simulink model "hd"  (R2016b)
settings: Solver=VariableStepAuto  StartTime=0.0  StopTime=totaltime  RelTol=1e-3
undefined symbols (not defined in the file or in its folder): A, N, st
libraries: xbsIndex_r4 x1, JTAGRuntimeCosim_r4 x1
settings Model: Creator=rm101  LastModifiedBy=rm101

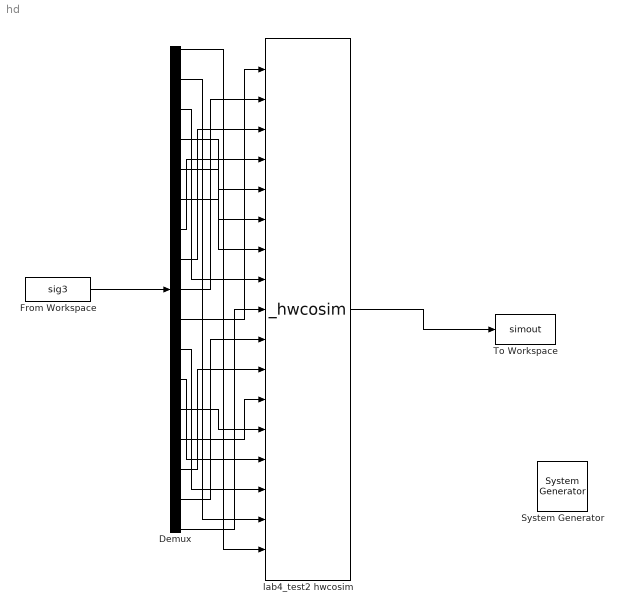
== system hd ==
  " System Generator" : xbsIndex_r4/ System Generator  Tag=genX  xilinxfamily=zynq  part=xc7z020  speed=-1  package=clg484  synthesis_tool=Vivado  clock_wrapper=Clock Enables  directory=C:/Users/rm101/Desktop/YG/Lab4_Matlab/gen  proj_type=Vivado  Synth_file=Vivado Synthesis Defaults  Impl_file=Vivado Implementation Defaults  testbench=off  simulink_period=st  sysclk_period=st*10e8  dcm_input_clock_period=10  incr_netlist=off  trim_vbits=Everywhere in SubSystem  dbl_ovrd=According to Block Masks  core_generation=According to Block Masks  run_coregen=off  deprecated_control=off  eval_field=0  block_type=sysgen
  Demux : Demux  Outputs=17
  From Workspace : FromWorkspace  VariableName=sig3  SampleTime=0  Interpolate=off  OutputAfterFinalValue=Holding final value
  To Workspace : ToWorkspace  VariableName=simout  SaveFormat=Timeseries  SampleTime=-1
  lab4_test2 hwcosim : JTAGRuntimeCosim_r4/_hwcosim  clkSrc=Single Stepped  hasCombinationalPath=on  bitfileName=C:\Users\rm101\Desktop\YG\Lab4_Matlab\gen\lab4_test2.bit  skipConfig=off  dispPartInfo=off  useZynqReconfigScript=on  cable=Auto Detect  speed=N/A  cablePort=N/A  cableLocation=Local  shareCable=off  design_xtable=|  engineDll=JTAGCosimEngine.dll  cableWaitTime=10  bscanPos=-1  IRLengths=[]  useWaitBox=1  hasBufgmux=on  Scheme=Cosim  useCmdProc=1  hasProc=0  useImpact=0  printLogFile=0  userChain=2  block_type=jtagcosim
      | {
      |     'clkWrapper' => 'lab4_test2',
      |     'burstMode' => false,
      |     'burstFifoDepth' => '1024',
      |     'shared_memories' => {},
      |     'clocksGcd' => 1,
      |     'device' => {
      |       'family' => 'zynq',
      |       'part' => 'xc7z020',
      |       'package' => 'clg484',
      |       'speed' => '-1',
      |     },
      |     'ports' => {
      |       'a9' => {
      |         'direction' => 'in',
      |         'width' => 8,
      |         'name' => 'a9',
      |         'period' => 1,
      |         'icon_text' => 'a9',
      |         'type' => 'Fix_8_6',
      |         'arithmetic_type' => 'xlSigned',
      |         'dat_file' => 'lab4_test2_subsystem_a9.dat',
      |         'bin_pt' => 6,
      |         'addr_offset' => 0,
      |         'bd_port_index' => 0,
      |       },
      |       'a8' => {
      |         'direction' => 'in',
      |         'width' => 8,
      |         'name' => 'a8',
      |         'period' => 1,
      |         'icon_text' => 'a8',
      |         'type' => 'Fix_8_6',
      |         'arithmetic_type' => 'xlSigned',
      |         'dat_file' => 'lab4_test2_subsystem_a8.dat',
      |         'bin_pt' => 6,
      |         'addr_offset' => 4,
      |         'bd_port_index' => 1,
      |       },
      |       'a7' => {
      |         'direction' => 'in',
      |         'width' => 8,
      |         'name' => 'a7',
      |         'period' => 1,
      |         'icon_text' => 'a7',
      |         'type' => 'Fix_8_6',
      |         'arithmetic_type' => 'xlSigned',
      |         'dat_file' => 'lab4_test2_subsystem_a7.dat',
      |         'bin_pt' => 6,
      |         'addr_offset' => 8,
      |         'bd_port_index' => 2,
      |       },
      |       'a6' => {
      |         'direction' => 'in',
      |         'width' => 8,
      |         'name' => 'a6',
      |         'period' => 1,
      |         'icon_text' => 'a6',
      |         'type' => 'Fix_8_6',
      |         'arithmetic_type' => 'xlSigned',
      |         'dat_file' => 'lab4_test2_subsystem_a6.dat',
      |         'bin_pt' => 6,
      |         'addr_offset' => 12,
      |         'bd_port_index' => 3,
      |       },
      |       'a5' => {
      |         'direction' => 'in',
      |         'width' => 8,
      |         'name' => 'a5',
      |         'period' => 1,
      |         'icon_text' => 'a5',
      |         'type' => 'Fix_8_6',
      |         'arithmetic_type' => 'xlSigned',
      |         'dat_file' => 'lab4_test2_subsystem_a5.dat',
      |         'bin_pt' => 6,
      |         'addr_offset' => 16,
      |         'bd_port_index' => 4,
      |       },
      |       'a4' => {
      |         'direction' => 'in',
      |         'width' => 8,
      |         'name' => 'a4',
      |         'period' => 1,
      |         'icon_text' => 'a4',
      |         'type' => 'Fix_8_6',
      |         'arithmetic_type' => 'xlSigned',
      |         'dat_file' => 'lab4_test2_subsystem_a4.dat',
      |         'bin_pt' => 6,
      |         'addr_offset' => 20,
      |         'bd_port_index' => 5,
      |       },
      |       'a3' => {
      |         'direction' => 'in',
      |         'width' => 8,
      |         'name' => 'a3',
      |         'period' => 1,
      |         'icon_text' => 'a3',
      |         'type' => 'Fix_8_6',
      |         'arithmetic_type' => 'xlSigned',
      |         'dat_file' => 'lab4_test2_subsystem_a3.dat',
      |         'bin_pt' => 6,
      |         'addr_offset' => 24,
      |         'bd_port_index' => 6,
      |       },
      |       'a2' => {
      |         'direction' => 'in',
      |         'width' => 8,
      |         'name' => 'a2',
      |         'period' => 1,
      |         'icon_text' => 'a2',
      |         'type' => 'Fix_8_6',
      |         'arithmetic_type' => 'xlSigned',
      |         'dat_file' => 'lab4_test2_subsystem_a2.dat',
      |         'bin_pt' => 6,
      |         'addr_offset' => 28,
      |         'bd_port_index' => 7,
      |       },
      |       'a16' => {
      |         'direction' => 'in',
      |         'width' => 8,
      |         'name' => 'a16',
      |         'period' => 1,
      |         'icon_text' => 'a16',
      |         'type' => 'Fix_8_6',
      |         'arithmetic_type' => 'xlSigned',
      |         'dat_file' => 'lab4_test2_subsystem_a16.dat',
      |         'bin_pt' => 6,
      |         'addr_offset' => 32,
      |         'bd_port_index' => 8,
      |       },
      |       'a15' => {
      |         'direction' => 'in',
      |         'width' => 8,
      |         'name' => 'a15',
      |         'period' => 1,
      |         'icon_text' => 'a15',
      |         'type' => 'Fix_8_6',
      |         'arithmetic_type' => 'xlSigned',
      |         'dat_file' => 'lab4_test2_subsystem_a15.dat',
      |         'bin_pt' => 6,
      |         'addr_offset' => 36,
      |         'bd_port_index' => 9,
      |       },
      |       'a14' => {
      |         'direction' => 'in',
      |         'width' => 8,
      |         'name' => 'a14',
      |         'period' => 1,
      |         'icon_text' => 'a14',
      |         'type' => 'Fix_8_6',
      |         'arithmetic_type' => 'xlSigned',
      |         'dat_file' => 'lab4_test2_subsystem_a14.dat',
      |         'bin_pt' => 6,
      |         'addr_offset' => 40,
      |         'bd_port_index' => 10,
      |       },
      |       'a13' => {
      |         'direction' => 'in',
      |         'width' => 8,
      |         'name' => 'a13',
      |         'period' => 1,
      |         'icon_text' => 'a13',
      |         'type' => 'Fix_8_6',
      |         'arithmetic_type' => 'xlSigned',
      |         'dat_file' => 'lab4_test2_subsystem_a13.dat',
      |         'bin_pt' => 6,
      |         'addr_offset' => 44,
      |         'bd_port_index' => 11,
      |       },
      |       'a12' => {
      |         'direction' => 'in',
      |         'width' => 8,
      |         'name' => 'a12',
      |         'period' => 1,
      |         'icon_text' => 'a12',
      |         'type' => 'Fix_8_6',
      |         'arithmetic_type' => 'xlSigned',
      |         'dat_file' => 'lab4_test2_subsystem_a12.dat',
      |         'bin_pt' => 6,
      |         'addr_offset' => 48,
      |         'bd_port_index' => 12,
      |       },
      |       'a11' => {
      |         'direction' => 'in',
      |         'width' => 8,
      |         'name' => 'a11',
      |         'period' => 1,
      |         'icon_text' => 'a11',
      |         'type' => 'Fix_8_6',
      |         'arithmetic_type' => 'xlSigned',
      |         'dat_file' => 'lab4_test2_subsystem_a11.dat',
      |         'bin_pt' => 6,
      |         'addr_offset' => 52,
      |         'bd_port_index' => 13,
      |       },
      |       'a10' => {
      |         'direction' => 'in',
      |         'width' => 8,
      |         'name' => 'a10',
      |         'period' => 1,
      |         'icon_text' => 'a10',
      |         'type' => 'Fix_8_6',
      |         'arithmetic_type' => 'xlSigned',
      |         'dat_file' => 'lab4_test2_subsystem_a10.dat',
      |         'bin_pt' => 6,
      |         'addr_offset' => 56,
      |         'bd_port_index' => 14,
      |       },
      |       'a1' => {
      |         'direction' => 'in',
      |         'width' => 8,
      |         'name' => 'a1',
      |         'period' => 1,
      |         'icon_text' => 'a1',
      |         'type' => 'Fix_8_6',
      |         'arithmetic_type' => 'xlSigned',
      |         'dat_file' => 'lab4_test2_subsystem_a1.dat',
      |         'bin_pt' => 6,
      |         'addr_offset' => 60,
      |         'bd_port_index' => 15,
      |       },
      |       'a' => {
      |         'direction' => 'in',
      |         'width' => 8,
      |         'name' => 'a',
      |         'period' => 1,
      |         'icon_text' => 'a',
      |         'type' => 'Fix_8_6',
      |         'arithmetic_type' => 'xlSigned',
      |         'dat_file' => 'lab4_test2_subsystem_a.dat',
      |         'bin_pt' => 6,
      |         'addr_offset' => 64,
      |         'bd_port_index' => 16,
      |       },
      |       'dout' => {
      |         'direction' => 'out',
      |         'width' => 17,
      |         'name' => 'dout',
      |         'period' => 1,
      |         'icon_text' => 'Dout',
      |         'type' => 'Fix_17_14',
      |         'arithmetic_type' => 'xlSigned',
      |         'dat_file' => 'lab4_test2_subsystem_dout.dat',
      |         'bin_pt' => 14,
      |         'addr_offset' => 68,
      |         'bd_port_index' => 0,
      |       },
      |     },
      |   }
  wires:
  lab4_test2 hwcosim/1 -> To Workspace/1
  From Workspace/1 -> Demux/1
  Demux/1 -> lab4_test2 hwcosim/17
  Demux/2 -> lab4_test2 hwcosim/16
  Demux/3 -> lab4_test2 hwcosim/8
  Demux/4 -> lab4_test2 hwcosim/7
  Demux/5 -> lab4_test2 hwcosim/6
  Demux/6 -> lab4_test2 hwcosim/5
  Demux/7 -> lab4_test2 hwcosim/4
  Demux/8 -> lab4_test2 hwcosim/3
  Demux/9 -> lab4_test2 hwcosim/2
  Demux/10 -> lab4_test2 hwcosim/1
  Demux/11 -> lab4_test2 hwcosim/15
  Demux/12 -> lab4_test2 hwcosim/14
  Demux/13 -> lab4_test2 hwcosim/13
  Demux/14 -> lab4_test2 hwcosim/12
  Demux/15 -> lab4_test2 hwcosim/11
  Demux/16 -> lab4_test2 hwcosim/10
  Demux/17 -> lab4_test2 hwcosim/9
